simulink subsystem "BATERIA_INVERSOR"  (R2020b)
settings: Solver=VariableStepAuto  StartTime=0.0  StopTime=10.0  RelTol=1e-3
undefined symbols (not defined in the file): Ion, Lithium, Ts
libraries: powerlib x34, powerlib_meascontrol x11, slpidlib x11, electricdrivelib x1, simulink x1
(part 1 of 2)
settings Model: Creator=JGC  LastModifiedBy=JGC

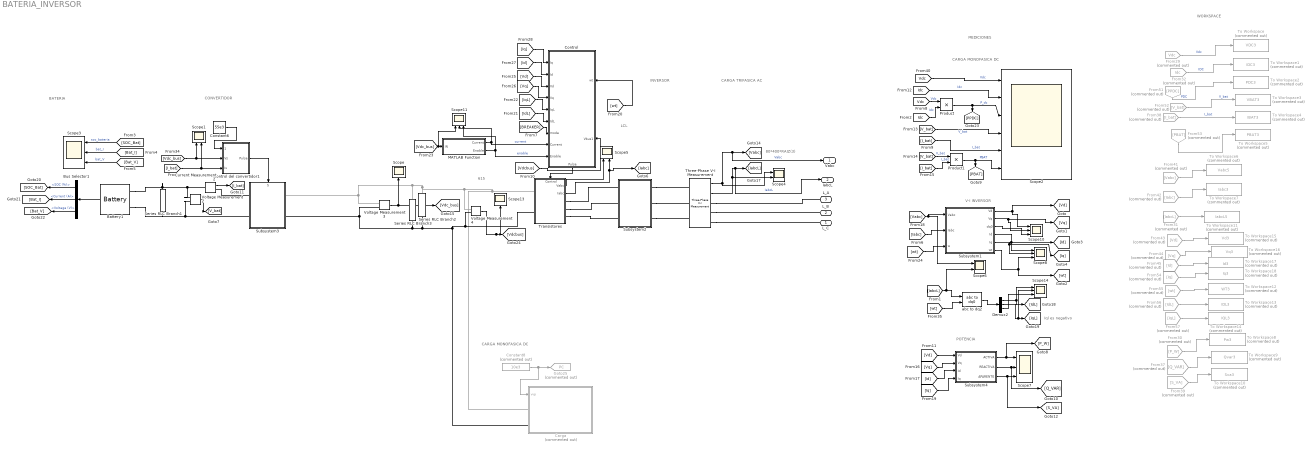
== system BATERIA_INVERSOR ==
  note: CARGA TRIFASICA AC
  note: LCL
  note: CARGA MONOFASICA DC
  note: BATERIA
  note: 80*400*RAIZ(3)
  note: 615
  note: CONVERTIDOR
  note: INVERSOR
  note: Iql es negativo
  note: V-I INVERSOR
  note: MEDICIONES
  note: CARGA MONOFASICA DC
  note: POTENCIA
  note: WORKSPACE
  Battery1 : electricdrivelib/Extra Sources/Battery  BatType=Lithium-Ion  ShowTempParam=off  ThermalPreset=no  ShowAgeParam=off  NomV=Battery.Nominal_voltage  NomQ=Battery.Rated_capacity  SOC=Battery.inicial_state_of_charge  Batt_Tr=Battery.response_time  PresetModel=on  MaxQ=200  MinV=384  FullV=595.9614  Dis_rate=86.9565  R=0.0256  Normal_OP=180.8696  expZone="[553.1576      9.826087]"  current=[6.5 7 100]  Units=Time  Tci=20  NomT=20  T2=-30  MaxQ2=4.8  FullV2=7.1  Normal_OP2=5.655  expZone2="[6.58           1]"  Rca=0.6  ti=2000  Dp=0  Neq0=0  Tsim=1e6  Ta1=25  Qeol=5.4*0.9  Reol=0.013333*1.2  Char_age=[2.3478, 3]  Dis_age=[2.3478, 10]  N1=1500  N2=10500  N3=1000  N4=1400  Ta2=45  N5=950
  Bus Selector1 : BusSelector  OutputSignals=SOC (%),Current (A),Voltage (V)
  Carga : Subsystem  Commented=on
  Constant6 : Constant  Value=55e3
  Constant8 : Constant  Commented=on  Value=10e3
  "Control " : Subsystem
      settings: PortSchema="{\"entries\":[{\"content\":{\"sides\":[{\"content\":{\"connectorIds\":[\"In1\",\"In2\",\"In3\",\"In4\",\"In5\",\"In6\",\"In7\",\"In8\",\"In9\"]},\"type\":\"ConnectorPlacement.EquallySpacedRectSide\",\"uuid\":\"040f479b-0063-4a97-945a-b7b76c14ccf9\"},{\"content\":{\"connectorIds\":[\"In10\",\"In11\"],\"side\":\"RIGHT\"},\"type\":\"ConnectorPlacement.EquallySpacedRectSide\",\"uuid\":\"48d15187-e0ba-47e4-acd1-e370322fb20d\"},{\"content\":{\"connectorIds\":[],\"side\":\"TOP\"},\"type\":\"ConnectorPlacement.EquallySpacedRectSide\",\"uuid\":\"c47ff363-741e-4c95-9660-92ffbbf0858a\"},{\"content\":{\"connectorIds\":[\"Out1\"],\"side\":\"BOTTOM\"},\"type\":\"ConnectorPlacement.EquallySpacedRectSide\",\"uuid\":\"eb550659-5dfa-48af-9c5b-3062ad81491f\"},{\"content\":{\"connectorIds\":[],\"side\":\"HIDDEN\"},\"type\":\"ConnectorPlacement.EquallySpacedRectSide\",\"uuid\":\"d4fe4439-474c-44ef-b2aa-466a1c380da3\"}]},\"type\":\"ConnectorPlacement.EquallySpacedConnector\",\"uuid\":\"b4b94fd9-d3fa-4033-a0eb-720d35d74a7d\"}],\"packageUris\":[\"http://schema.mathworks.com/mf0/Connector/R2020b\"],\"version\":\"1.0\"}"
  Control del convertidor1 : Subsystem
  Current Measurement2 : powerlib/Measurements/Current Measurement  PhasorSimulation=off  OutputType=Complex  PSBequivalent=0
  Demux2 : Demux  Outputs=3
  From29 : From  Commented=on  GotoTag=Vdc
  From30 : From  Commented=on  GotoTag=P_W
  From31 : From  Commented=on  GotoTag=IabcL
  From32 : From  Commented=on  GotoTag=Idc
  From37 : From  Commented=on  GotoTag=Q_VAR
  From38 : From  Commented=on  GotoTag=I_bat
  From39 : From  Commented=on  GotoTag=S_VA
  From41 : From  Commented=on  GotoTag=Vabc
  From42 : From  Commented=on  GotoTag=Iabc
  From43 : From  Commented=on  GotoTag=Vd
  From44 : From  Commented=on  GotoTag=Vq
  From45 : From  Commented=on  GotoTag=Id
  From51 : From  Commented=on  GotoTag=PPDC
  From52 : From  Commented=on  GotoTag=V_bat
  From53 : From  Commented=on  GotoTag=PBAT
  From54 : From  Commented=on  GotoTag=Iq
  From55 : From  Commented=on  GotoTag=wt
  From56 : From  Commented=on  GotoTag=IdL
  From57 : From  Commented=on  GotoTag=IqL
  Goto25 : Goto  Commented=on  GotoTag=PC  TagVisibility=global
  MATLAB Function : MATLAB Function  TreatAsAtomicUnit=on
  Product : Product
  Product1 : Product
  Scope : Scope
  Scope{1,4..6} (4 alike) : Scope  NumInputPorts=2
  Scope{3,7..8,10..11,14} (6 alike) : Scope  NumInputPorts=3
  Scope13 : Scope
  Scope2 : Scope  NumInputPorts=6
  Series RLC Branch1 : powerlib/Elements/Series RLC Branch  LConnTagsString=__new0  RConnTagsString=__new0  BranchType=RC  Resistance=0.3  Inductance=1e-3  SetiL0=off  InitialCurrent=0  Capacitance=1e-6  Setx0=on  InitialVoltage=512  Measurements=None
  Series RLC Branch2 : powerlib/Elements/Series RLC Branch  LConnTagsString=__new0  RConnTagsString=__new0  BranchType=C  Resistance=0.2  Inductance=1e-3  SetiL0=off  InitialCurrent=0  Capacitance=1000e-6  Setx0=on  InitialVoltage=550  Measurements=None
  Series RLC Branch3 : powerlib/Elements/Series RLC Branch  LConnTagsString=__new0  RConnTagsString=__new0  BranchType=R  Resistance=38  Inductance=1e-3  SetiL0=off  InitialCurrent=0  Capacitance=1e-6  Setx0=on  InitialVoltage=512  Measurements=None
  Subsystem1 : Subsystem
  Subsystem2 : Subsystem
  Subsystem3 : Subsystem
      settings: PortSchema="{\"entries\":[{\"content\":{\"sides\":[{\"content\":{\"connectorIds\":[\"LConn1\",\"LConn2\"]},\"type\":\"ConnectorPlacement.EquallySpacedRectSide\",\"uuid\":\"7a980847-0fd3-4a52-ae22-59cd2a1ed559\"},{\"content\":{\"connectorIds\":[\"RConn1\",\"RConn2\"],\"side\":\"RIGHT\"},\"type\":\"ConnectorPlacement.EquallySpacedRectSide\",\"uuid\":\"85effeeb-73a6-4b0a-b51b-5eb0082317ff\"},{\"content\":{\"connectorIds\":[\"In1\"],\"side\":\"TOP\"},\"type\":\"ConnectorPlacement.EquallySpacedRectSide\",\"uuid\":\"eb55fae0-79ad-414f-ab96-49c332138803\"},{\"content\":{\"connectorIds\":[],\"side\":\"BOTTOM\"},\"type\":\"ConnectorPlacement.EquallySpacedRectSide\",\"uuid\":\"1fd972ff-419a-4657-8ea4-57d89be2b868\"}]},\"type\":\"ConnectorPlacement.EquallySpacedConnector\",\"uuid\":\"1807473d-fd42-44e0-a7e4-668a7bf21429\"}],\"packageUris\":[\"http://schema.mathworks.com/mf0/Connector/R2020b\"],\"version\":\"1.0\"}"
  Subsystem4 : Subsystem
  Three-Phase V-I Measurement : powerlib/Measurements/Three-Phase V-I Measurement  VoltageMeasurement=phase-to-phase  SetLabelV=off  LabelV=Vabc  Vpu=off  VpuLL=off  CurrentMeasurement=yes  SetLabelI=off  LabelI=Iabc  Ipu=off  Pbase=100e6  Vbase=500e3  OutputType=Complex  PhasorSimulation=off  PSBequivalent=0
  To Workspace : ToWorkspace  Commented=on  VariableName=VDC3  SaveFormat=Timeseries  SampleTime=-1
  To Workspace1 : ToWorkspace  Commented=on  VariableName=IDC3  SaveFormat=Timeseries  SampleTime=-1
  To Workspace10 : ToWorkspace  Commented=on  VariableName=Sva3  SaveFormat=Timeseries  SampleTime=-1
  To Workspace11 : ToWorkspace  Commented=on  VariableName=IabcL5  SaveFormat=Structure With Time  SampleTime=-1
  To Workspace12 : ToWorkspace  Commented=on  VariableName=WT3  SaveFormat=Timeseries  SampleTime=-1
  To Workspace13 : ToWorkspace  Commented=on  VariableName=IDL3  SaveFormat=Timeseries  SampleTime=-1
  To Workspace14 : ToWorkspace  Commented=on  VariableName=IQL3  SaveFormat=Timeseries  SampleTime=-1
  To Workspace15 : ToWorkspace  Commented=on  VariableName=Vd3  SaveFormat=Timeseries  SampleTime=-1
  To Workspace16 : ToWorkspace  Commented=on  VariableName=Vq3  SaveFormat=Timeseries  SampleTime=-1
  To Workspace17 : ToWorkspace  Commented=on  VariableName=Id3  SaveFormat=Timeseries  SampleTime=-1
  To Workspace18 : ToWorkspace  Commented=on  VariableName=Iq3  SaveFormat=Timeseries  SampleTime=-1
  To Workspace2 : ToWorkspace  Commented=on  VariableName=PDC3  SaveFormat=Timeseries  SampleTime=-1
  To Workspace3 : ToWorkspace  Commented=on  VariableName=VBAT3  SaveFormat=Timeseries  SampleTime=-1
  To Workspace4 : ToWorkspace  Commented=on  VariableName=IBAT3  SaveFormat=Timeseries  SampleTime=-1
  To Workspace5 : ToWorkspace  Commented=on  VariableName=PBAT3  SaveFormat=Timeseries  SampleTime=-1
  To Workspace6 : ToWorkspace  Commented=on  VariableName=Vabc5  SaveFormat=Structure With Time  SampleTime=-1
  To Workspace7 : ToWorkspace  Commented=on  VariableName=Iabc3  SaveFormat=Timeseries  SampleTime=-1
  To Workspace8 : ToWorkspace  Commented=on  VariableName=Pw3  SaveFormat=Timeseries  SampleTime=-1
  To Workspace9 : ToWorkspace  Commented=on  VariableName=Qvar3  SaveFormat=Timeseries  SampleTime=-1
  Transistores : Subsystem
      settings: PortSchema="{\"entries\":[{\"content\":{\"sides\":[{\"content\":{\"connectorIds\":[\"LConn1\",\"LConn2\"]},\"type\":\"ConnectorPlacement.EquallySpacedRectSide\",\"uuid\":\"4b4a90af-a54c-4879-a767-640ef5f3fcb3\"},{\"content\":{\"connectorIds\":[\"Out1\",\"Out2\",\"RConn1\",\"RConn2\",\"RConn3\"],\"side\":\"RIGHT\"},\"type\":\"ConnectorPlacement.EquallySpacedRectSide\",\"uuid\":\"9175716d-9f9b-4229-800b-ed18d0bc4919\"},{\"content\":{\"connectorIds\":[\"In1\"],\"side\":\"TOP\"},\"type\":\"ConnectorPlacement.EquallySpacedRectSide\",\"uuid\":\"ad8bb3e4-0cf0-4c72-aeb3-553776322e14\"},{\"content\":{\"connectorIds\":[],\"side\":\"HIDDEN\"},\"type\":\"ConnectorPlacement.EquallySpacedRectSide\",\"uuid\":\"389b5ba2-67e8-44c1-bbe9-0320a382984d\"}]},\"type\":\"ConnectorPlacement.EquallySpacedConnector\",\"uuid\":\"7a2ee168-b262-4afb-be64-1e845efa873f\"}],\"packageUris\":[\"http://schema.mathworks.com/mf0/Connector/R2020b\"],\"version\":\"1.0\"}"
  Voltage Measurement2 : powerlib/Measurements/Voltage Measurement  PhasorSimulation=off  OutputType=Complex  PSBequivalent=0
  Voltage Measurement3 : powerlib/Measurements/Voltage Measurement  PhasorSimulation=off  OutputType=Complex  PSBequivalent=0
  Voltage Measurement4 : powerlib/Measurements/Voltage Measurement  PhasorSimulation=off  OutputType=Complex  PSBequivalent=0
  abc to dq2 : powerlib_meascontrol/Transformations/abc to dq0  Alignment=90 degrees behind phase A axis
  L_C : PMIOPort  Side=Right
  L_B : PMIOPort  Port=2  Side=Right
  L_A : PMIOPort  Port=3  Side=Right
  Vabc : Outport
  IabcL : Outport  Port=2
  wires:
  Current Measurement2/1 -> [I_bat]
  Voltage Measurement2/1 -> [V_bat]
  Transistores/1(Vabc) -> Scope5/1
  Control del convertidor1/1(Pulse) -> Subsystem3/1(S)
  [Bat_V] -> Scope3/3  "bat_V"
  Transistores/2(Iabc) -> Scope5/2, [Iabc]
  Three-Phase V-I Measurement/2 -> Scope4/2, [IabcL], IabcL/1  "IabcL"
  Constant6/1 -> Control del convertidor1/1(Pot_ref)
  [Bat_I] -> Scope3/2  "bat_I"
  Three-Phase V-I Measurement/1 -> Scope4/1, [Vabc], Vabc/1  "Vabc"
  "Control "/1(Pulse) -> Transistores/1(Control)
  MATLAB Function/2(Enable) -> "Control "/9(Enable), Scope11/3  "enable"
  Battery1/1 -> Bus Selector1/1
  [Vdc_bus] -> Control del convertidor1/2(Vs), Scope1/1
  [I_bat] -> Scope1/2, Control del convertidor1/3(Is)
  MATLAB Function/1(Current) -> "Control "/8(Current), Scope11/2  "current"
  Bus Selector1/2 -> [Bat_I]  "<Current (A)>"
  Constant8/1 -> Carga/1(vvp), Goto25/1
  Bus Selector1/1 -> [SOC_Bat]  "<SOC (%)>"
  Voltage Measurement3/1 -> Scope/1, [Vdc_bus]
  [SOC_Bat] -> Scope3/1  "soc_bateria"
  Bus Selector1/3 -> [Bat_V]  "<Voltage (V)>"
  Voltage Measurement4/1 -> [Vdcbus], Scope13/1
  [Vdc_bus] -> MATLAB Function/1(IN), Scope11/1
  [Vdcbus] -> "Control "/11(Vbus1)
  [BREAKER] -> "Control "/7(mode)
  Demux2/1 -> Scope14/1, [IdL]
  [I_bat] -> Product1/2  "I_bat"
  [I_bat] -> Scope2/5  "I_bat"
  Demux2/2 -> [IqL], Scope14/2
  Subsystem1/2(Vq) -> [Vq], Scope10/2
  abc to dq2/1 -> Demux2/1
  [Vdc] -> Scope2/1  "Vdc"
  Subsystem4/1(ACTIVA) -> Scope7/1, [P_W]
  [Idc] -> Scope2/2  "Idc"
  Subsystem1/5(Iq) -> [Iq], Scope8/2
  [V_bat] -> Product1/1  "V_bat"
  [IabcL] -> abc to dq2/1, Scope6/2
  [V_bat] -> Scope2/4  "V_bat"
  Subsystem1/6(wt) -> Scope8/3, [wt]
  [Vdc] -> Product/1  "Vdc"
  Product1/1 -> [PBAT], Scope2/6  "PBAT"
  [Iabc] -> Subsystem1/2(Iabc)
  Subsystem1/1(Vd) -> [Vd], Scope10/1
  Product/1 -> [PPDC], Scope2/3  "P_dc"
  [wt] -> abc to dq2/2
  [Idc] -> Product/2  "Idc"
  Subsystem1/4(Id) -> Scope8/1, [Id]
  Demux2/3 -> Scope14/3
  [Vabc] -> Subsystem1/1(Vabc), Scope6/1
  Subsystem4/3(APARENTE) -> Scope7/3, [S_VA]
  Subsystem1/3(dq0) -> Scope10/3
  Subsystem4/2(REACTIVA) -> Scope7/2, [Q_VAR]
  [Vd] -> Subsystem4/1(Vd)
  [Vq] -> Subsystem4/2(Vq)
  [Id] -> Subsystem4/3(Id)
  [Iq] -> Subsystem4/4(Iq)
  [wt] -> "Control "/10(wt)
  [IdL] -> "Control "/6(IdL)
  [IqL] -> "Control "/5(IqL)
  [wt] -> Subsystem1/3(w)
  [Vd] -> "Control "/3(Vd)
  [Vq] -> "Control "/4(Vq)
  [Id] -> "Control "/2(Id)
  [Iq] -> "Control "/1(Iq)
  From56/1 -> To Workspace13/1
  From45/1 -> To Workspace17/1
  From31/1 -> To Workspace11/1
  From54/1 -> To Workspace18/1
  From51/1 -> To Workspace2/1  "PDC"
  From39/1 -> To Workspace10/1
  From43/1 -> To Workspace15/1
  From53/1 -> To Workspace5/1
  From52/1 -> To Workspace3/1  "V_bat"
  From37/1 -> To Workspace9/1
  From41/1 -> To Workspace6/1
  From42/1 -> To Workspace7/1
  From38/1 -> To Workspace4/1  "I_bat"
  From57/1 -> To Workspace14/1
  From29/1 -> To Workspace/1  "Vdc"
  From30/1 -> To Workspace8/1
  From32/1 -> To Workspace1/1  "IDC"
  From55/1 -> To Workspace12/1
  From44/1 -> To Workspace16/1
  connections:
  Carga/LConn1 -- Voltage Measurement3/LConn1 -- Subsystem3/RConn1 -- Series RLC Branch3/LConn1 -- Series RLC Branch2/LConn1 -- Voltage Measurement4/LConn1 -- Transistores/LConn1
  Series RLC Branch1/LConn1 -- Current Measurement2/LConn1 -- Voltage Measurement2/LConn1 -- Battery1/LConn1
  Transistores/LConn2 -- Voltage Measurement3/LConn2 -- Subsystem3/RConn2 -- Series RLC Branch3/RConn1 -- Series RLC Branch2/RConn1 -- Carga/LConn2 -- Voltage Measurement4/LConn2
  Subsystem3/LConn2 -- Series RLC Branch1/RConn1 -- Battery1/LConn2 -- Voltage Measurement2/LConn2
  Subsystem3/LConn1 -- Current Measurement2/RConn1
  Three-Phase V-I Measurement/RConn2 -- L_B/RConn1
  Subsystem2/LConn2 -- Three-Phase V-I Measurement/LConn2
  Three-Phase V-I Measurement/RConn1 -- L_A/RConn1
  Three-Phase V-I Measurement/RConn3 -- L_C/RConn1
  Transistores/RConn2 -- Subsystem2/RConn2
  Subsystem2/LConn3 -- Three-Phase V-I Measurement/LConn3
  Subsystem2/LConn1 -- Three-Phase V-I Measurement/LConn1
  Transistores/RConn3 -- Subsystem2/RConn3
  Transistores/RConn1 -- Subsystem2/RConn1

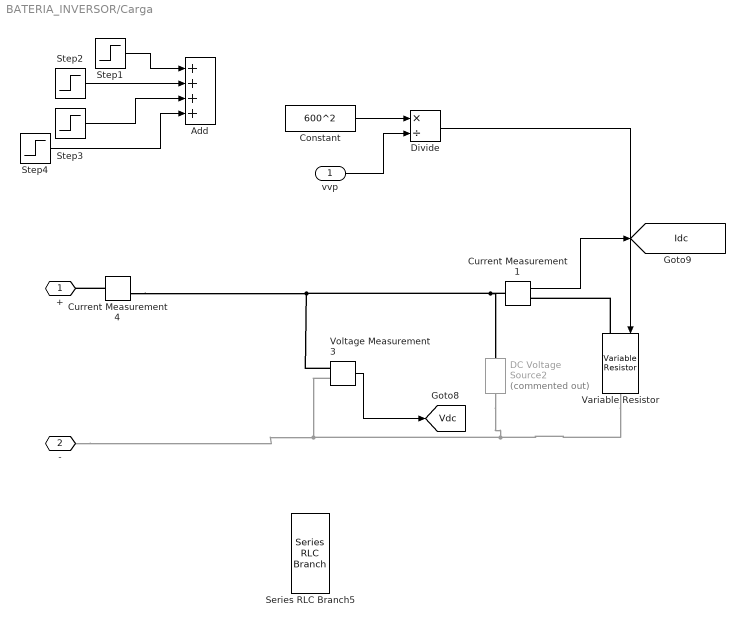
== system BATERIA_INVERSOR/Carga ==
  vvp : Inport
  Add : Sum  Inputs=++++
  Constant : Constant  Value=600^2
  Current Measurement1 : powerlib/Measurements/Current Measurement  PhasorSimulation=off  OutputType=Complex  PSBequivalent=0
  Current Measurement4 : powerlib/Measurements/Current Measurement  PhasorSimulation=off  OutputType=Complex  PSBequivalent=0
  DC Voltage Source2 : powerlib/Electrical Sources/DC Voltage Source  Commented=on  Amplitude=800  Measurements=None
  Divide : Product  Inputs=*/
  Series RLC Branch5 : powerlib/Elements/Series RLC Branch  LConnTagsString=__new0  RConnTagsString=__new0  BranchType=C  Resistance=0.2  Inductance=1e-3  SetiL0=off  InitialCurrent=0  Capacitance=300e-6  Setx0=on  InitialVoltage=512  Measurements=None
  Step1 : Step  After=5000  SampleTime=0
  Step2 : Step  Time=2  After=-7500  SampleTime=0
  Step3 : Step  Time=3  After=10000  SampleTime=0
  Step4 : Step  Time=4  After=-7500  SampleTime=0
  Variable Resistor : powerlib/Elements/Variable Resistor  Rabsmin=1e-3
      settings: SourceProductBaseCode=PS
  Voltage Measurement3 : powerlib/Measurements/Voltage Measurement  PhasorSimulation=off  OutputType=Complex  PSBequivalent=0
  + : PMIOPort  Side=Left
  - : PMIOPort  Port=2  Side=Left
  tag scope: Idc=global, Vdc=global
  wires:
  vvp/1 -> Divide/2
  Current Measurement1/1 -> [Idc]
  Step4/1 -> Add/4
  Step3/1 -> Add/3
  Step2/1 -> Add/2
  Step1/1 -> Add/1
  Divide/1 -> Variable Resistor/1
  Constant/1 -> Divide/1
  Voltage Measurement3/1 -> [Vdc]
  connections:
  Current Measurement1/LConn1 -- DC Voltage Source2/RConn1 -- Voltage Measurement3/LConn1 -- Current Measurement4/RConn1
  Variable Resistor/LConn1 -- Current Measurement1/RConn1
  Current Measurement4/LConn1 -- +/RConn1
  DC Voltage Source2/LConn1 -- Variable Resistor/RConn1 -- -/RConn1 -- Voltage Measurement3/LConn2

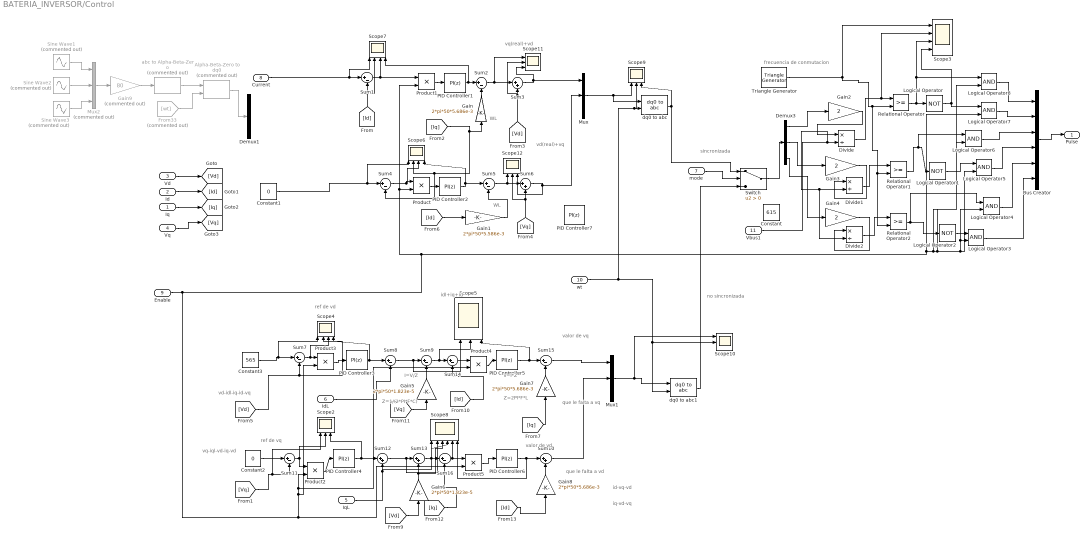
== system BATERIA_INVERSOR/Control  ==
  note: v=I*Z
  note: Z=2PI*F*L
  note: vd-idl-iq-id-vq
  note: ref de vq
  note: que le falta a vd
  note: ref de vd
  note: que le falta a vq
  note: valor de vq
  note: iq-vd-vq
  note: valor de vd
  note: vq-iql-vd-iq-vd
  note: I=V/Z
  note: Z=1/(2*PI*F*C)
  note: id-vq-vd
  note: idl+iq+id
  note: vq(real)+vd
  note: vd(real)+vq
  note: WL
  note: WL
  note: frecuencia de conmutacion
  note: no sincronizada
  note: sincronizada
  Iq : Inport
  Id : Inport  Port=2
  Vd : Inport  Port=3
  Vq : Inport  Port=4
  IqL : Inport  Port=5
  IdL : Inport  Port=6
  mode : Inport  Port=7
  Current : Inport  Port=8
  Enable : Inport  Port=9
  wt : Inport  Port=10
  Vbus1 : Inport  Port=11
  Alpha-Beta-Zero to dq0 : powerlib_meascontrol/Transformations/Alpha-Beta-Zero to dq0  Commented=on  Alignment=90 degrees behind phase A axis
  Bus Creator : BusCreator  Inputs=6
  Constant : Constant  Value=615
  Constant1 : Constant  Value=0
  Constant2 : Constant  Value=0
  Constant3 : Constant  Value=565
  Demux1 : Demux  Outputs=3
  Demux3 : Demux  Outputs=3
  Divide : Product  Inputs=*/
  Divide1 : Product  Inputs=*/
  Divide2 : Product  Inputs=*/
  From33 : From  Commented=on  GotoTag=wt  TagVisibility=global
  Gain : Gain  Gain=2*pi*50*5.686e-3
  Gain1 : Gain  Gain=2*pi*50*5.586e-3
  Gain2 : Gain  Gain=2
  Gain3 : Gain  Gain=2
  Gain4 : Gain  Gain=2
  Gain5 : Gain  Gain=2*pi*50*1.823e-5
  Gain6 : Gain  Gain=2*pi*50*1.823e-5
  Gain7 : Gain  Gain=2*pi*50*5.686e-3
  Gain8 : Gain  Gain=2*pi*50*5.686e-3
  Gain9 : Gain  Commented=on  Gain=80
  Logical Operator : Logic  Operator=NOT  AllPortsSameDT=off  OutDataTypeStr=boolean
  Logical Operator1 : Logic  Operator=NOT  AllPortsSameDT=off  OutDataTypeStr=boolean
  Logical Operator2 : Logic  Operator=NOT  AllPortsSameDT=off  OutDataTypeStr=boolean
  Logical Operator{3..8} (6 alike) : Logic  AllPortsSameDT=off  OutDataTypeStr=boolean
  Mux : Mux  Inputs=3
  Mux1 : Mux  Inputs=3
  Mux2 : Mux  Commented=on  Inputs=3
  PID Controller1 : slpidlib/PID Controller  Controller=PI  Form=Parallel  TimeDomain=Discrete-time  UseExternalTs=off  SampleTime=Ts  IntegratorMethod=Forward Euler  FilterMethod=Forward Euler  ControllerParametersSource=internal  P=60  I=0  D=0  UseFilter=on  N=100  TunerSelectOption=Transfer Function Based (PID Tuner App)  InitialConditionSource=internal  InitialConditionForIntegrator=0  InitialConditionForFilter=0  DifferentiatorICPrevScaledInput=0  ExternalReset=none  TrackingMode=off  Kt=1  LimitOutput=off  SatLimitsSource=internal  UpperSaturationLimit=inf  LowerSaturationLimit=-inf  LinearizeAsGain=on  AntiWindupMode=none  Kb=1  POutMin=[]  POutMax=[]  IOutMin=[]  IOutMax=[]  DOutMin=[]  DOutMax=[]  NOutMin=[]  NOutMax=[]  SumOutMin=[]  SumOutMax=[]  SaturationOutMin=[]  SaturationOutMax=[]  PParamMin=[]  PParamMax=[]  IParamMin=[]  IParamMax=[]  DParamMin=[]  DParamMax=[]  NParamMin=[]  NParamMax=[]  KbParamMin=[]  KbParamMax=[]  KtParamMin=[]  KtParamMax=[]  KbOutMin=[]  KbOutMax=[]  KtOutMin=[]  KtOutMax=[]  IntegratorOutMin=[]  IntegratorOutMax=[]  FilterOutMin=[]  FilterOutMax=[]  SumI1OutMin=[]  SumI1OutMax=[]  SumI2OutMin=[]  SumI2OutMax=[]  SumI3OutMin=[]  SumI3OutMax=[]  SumI4OutMin=[]  SumI4OutMax=[]  SumDOutMin=[]  SumDOutMax=[]  DifferentiatorOutMin=[]  DifferentiatorOutMax=[]  FilterDiffOutCoefMin=[]  FilterDiffOutCoefMax=[]  ReciprocalOutMin=[]  ReciprocalOutMax=[]  SumDenOutMin=[]  SumDenOutMax=[]  SumNumOutMin=[]  SumNumOutMax=[]  DivideOutMin=[]  DivideOutMax=[]  UdiffTsProdOutMin=[]  UdiffTsProdOutMax=[]  NTsProdOutMin=[]  NTsProdOutMax=[]  UintegralTsProdOutMin=[]  UintegralTsProdOutMax=[]  UngainTsProdOutMin=[]  UngainTsProdOutMax=[]  IntegratorContinuousStateAttributes=''  IntegratorStateMustResolveToSignalObject=off  IntegratorRTWStateStorageClass=Auto  FilterContinuousStateAttributes=''  FilterStateMustResolveToSignalObject=off  FilterRTWStateStorageClass=Auto  ParallelPVariant=InternalParameters  IdealPVariant=Disabled  IVariant=InternalParameters  DVariant=Disabled  IntegratorVariant=Discrete  SatVariant=Disabled  AWVariant=Passthrough  PCopyVariant=Disabled  TRVariant=Disabled  FdbkBlocksVariant=Forward  IdealPFdbkVariant=Disabled  SatFdbkVariant=Disabled  DerivativeFilterVariant=Disabled  NVariant=Disabled  NCopyVariant=Disabled_SignalSpec  FilterICVariant=Disabled  IntegratorICVariant=InternalICs  ExternalResetVariant=Disabled  TRSumVariant=Passthrough  SumFdbkVariant=Disabled  SumVariant=Sum_PI  TsampFilterVariant=InternalTs  TsampNgainVariant=Passthrough  TsampIntegralVariant=Passthrough  ExternalSaturationOutDataTypeStr=Inherit: Same as second input
  PID Controller2 : slpidlib/PID Controller  Controller=PI  Form=Parallel  TimeDomain=Discrete-time  UseExternalTs=off  SampleTime=Ts  IntegratorMethod=Forward Euler  FilterMethod=Forward Euler  ControllerParametersSource=internal  P=70  I=10  D=0  UseFilter=on  N=100  TunerSelectOption=Transfer Function Based (PID Tuner App)  InitialConditionSource=internal  InitialConditionForIntegrator=0  InitialConditionForFilter=0  DifferentiatorICPrevScaledInput=0  ExternalReset=none  TrackingMode=off  Kt=1  LimitOutput=off  SatLimitsSource=internal  UpperSaturationLimit=inf  LowerSaturationLimit=-inf  LinearizeAsGain=on  AntiWindupMode=none  Kb=1  POutMin=[]  POutMax=[]  IOutMin=[]  IOutMax=[]  DOutMin=[]  DOutMax=[]  NOutMin=[]  NOutMax=[]  SumOutMin=[]  SumOutMax=[]  SaturationOutMin=[]  SaturationOutMax=[]  PParamMin=[]  PParamMax=[]  IParamMin=[]  IParamMax=[]  DParamMin=[]  DParamMax=[]  NParamMin=[]  NParamMax=[]  KbParamMin=[]  KbParamMax=[]  KtParamMin=[]  KtParamMax=[]  KbOutMin=[]  KbOutMax=[]  KtOutMin=[]  KtOutMax=[]  IntegratorOutMin=[]  IntegratorOutMax=[]  FilterOutMin=[]  FilterOutMax=[]  SumI1OutMin=[]  SumI1OutMax=[]  SumI2OutMin=[]  SumI2OutMax=[]  SumI3OutMin=[]  SumI3OutMax=[]  SumI4OutMin=[]  SumI4OutMax=[]  SumDOutMin=[]  SumDOutMax=[]  DifferentiatorOutMin=[]  DifferentiatorOutMax=[]  FilterDiffOutCoefMin=[]  FilterDiffOutCoefMax=[]  ReciprocalOutMin=[]  ReciprocalOutMax=[]  SumDenOutMin=[]  SumDenOutMax=[]  SumNumOutMin=[]  SumNumOutMax=[]  DivideOutMin=[]  DivideOutMax=[]  UdiffTsProdOutMin=[]  UdiffTsProdOutMax=[]  NTsProdOutMin=[]  NTsProdOutMax=[]  UintegralTsProdOutMin=[]  UintegralTsProdOutMax=[]  UngainTsProdOutMin=[]  UngainTsProdOutMax=[]  IntegratorContinuousStateAttributes=''  IntegratorStateMustResolveToSignalObject=off  IntegratorRTWStateStorageClass=Auto  FilterContinuousStateAttributes=''  FilterStateMustResolveToSignalObject=off  FilterRTWStateStorageClass=Auto  ParallelPVariant=InternalParameters  IdealPVariant=Disabled  IVariant=InternalParameters  DVariant=Disabled  IntegratorVariant=Discrete  SatVariant=Disabled  AWVariant=Passthrough  PCopyVariant=Disabled  TRVariant=Disabled  FdbkBlocksVariant=Forward  IdealPFdbkVariant=Disabled  SatFdbkVariant=Disabled  DerivativeFilterVariant=Disabled  NVariant=Disabled  NCopyVariant=Disabled_SignalSpec  FilterICVariant=Disabled  IntegratorICVariant=InternalICs  ExternalResetVariant=Disabled  TRSumVariant=Passthrough  SumFdbkVariant=Disabled  SumVariant=Sum_PI  TsampFilterVariant=InternalTs  TsampNgainVariant=Passthrough  TsampIntegralVariant=Passthrough  ExternalSaturationOutDataTypeStr=Inherit: Same as second input
  PID Controller3 : slpidlib/PID Controller  Controller=PI  Form=Parallel  TimeDomain=Discrete-time  UseExternalTs=off  SampleTime=Ts  IntegratorMethod=Forward Euler  FilterMethod=Forward Euler  ControllerParametersSource=internal  P=1  I=180  D=0  UseFilter=on  N=100  TunerSelectOption=Transfer Function Based (PID Tuner App)  InitialConditionSource=internal  InitialConditionForIntegrator=0  InitialConditionForFilter=0  DifferentiatorICPrevScaledInput=0  ExternalReset=none  TrackingMode=off  Kt=1  LimitOutput=off  SatLimitsSource=internal  UpperSaturationLimit=inf  LowerSaturationLimit=-inf  LinearizeAsGain=on  AntiWindupMode=none  Kb=1  POutMin=[]  POutMax=[]  IOutMin=[]  IOutMax=[]  DOutMin=[]  DOutMax=[]  NOutMin=[]  NOutMax=[]  SumOutMin=[]  SumOutMax=[]  SaturationOutMin=[]  SaturationOutMax=[]  PParamMin=[]  PParamMax=[]  IParamMin=[]  IParamMax=[]  DParamMin=[]  DParamMax=[]  NParamMin=[]  NParamMax=[]  KbParamMin=[]  KbParamMax=[]  KtParamMin=[]  KtParamMax=[]  KbOutMin=[]  KbOutMax=[]  KtOutMin=[]  KtOutMax=[]  IntegratorOutMin=[]  IntegratorOutMax=[]  FilterOutMin=[]  FilterOutMax=[]  SumI1OutMin=[]  SumI1OutMax=[]  SumI2OutMin=[]  SumI2OutMax=[]  SumI3OutMin=[]  SumI3OutMax=[]  SumI4OutMin=[]  SumI4OutMax=[]  SumDOutMin=[]  SumDOutMax=[]  DifferentiatorOutMin=[]  DifferentiatorOutMax=[]  FilterDiffOutCoefMin=[]  FilterDiffOutCoefMax=[]  ReciprocalOutMin=[]  ReciprocalOutMax=[]  SumDenOutMin=[]  SumDenOutMax=[]  SumNumOutMin=[]  SumNumOutMax=[]  DivideOutMin=[]  DivideOutMax=[]  UdiffTsProdOutMin=[]  UdiffTsProdOutMax=[]  NTsProdOutMin=[]  NTsProdOutMax=[]  UintegralTsProdOutMin=[]  UintegralTsProdOutMax=[]  UngainTsProdOutMin=[]  UngainTsProdOutMax=[]  IntegratorContinuousStateAttributes=''  IntegratorStateMustResolveToSignalObject=off  IntegratorRTWStateStorageClass=Auto  FilterContinuousStateAttributes=''  FilterStateMustResolveToSignalObject=off  FilterRTWStateStorageClass=Auto  ParallelPVariant=InternalParameters  IdealPVariant=Disabled  IVariant=InternalParameters  DVariant=Disabled  IntegratorVariant=Discrete  SatVariant=Disabled  AWVariant=Passthrough  PCopyVariant=Disabled  TRVariant=Disabled  FdbkBlocksVariant=Forward  IdealPFdbkVariant=Disabled  SatFdbkVariant=Disabled  DerivativeFilterVariant=Disabled  NVariant=Disabled  NCopyVariant=Disabled_SignalSpec  FilterICVariant=Disabled  IntegratorICVariant=InternalICs  ExternalResetVariant=Disabled  TRSumVariant=Passthrough  SumFdbkVariant=Disabled  SumVariant=Sum_PI  TsampFilterVariant=InternalTs  TsampNgainVariant=Passthrough  TsampIntegralVariant=Passthrough  ExternalSaturationOutDataTypeStr=Inherit: Same as second input
  PID Controller4 : slpidlib/PID Controller  Controller=PI  Form=Parallel  TimeDomain=Discrete-time  UseExternalTs=off  SampleTime=Ts  IntegratorMethod=Forward Euler  FilterMethod=Forward Euler  ControllerParametersSource=internal  P=1  I=180  D=0  UseFilter=on  N=100  TunerSelectOption=Transfer Function Based (PID Tuner App)  InitialConditionSource=internal  InitialConditionForIntegrator=0  InitialConditionForFilter=0  DifferentiatorICPrevScaledInput=0  ExternalReset=none  TrackingMode=off  Kt=1  LimitOutput=off  SatLimitsSource=internal  UpperSaturationLimit=inf  LowerSaturationLimit=-inf  LinearizeAsGain=on  AntiWindupMode=none  Kb=1  POutMin=[]  POutMax=[]  IOutMin=[]  IOutMax=[]  DOutMin=[]  DOutMax=[]  NOutMin=[]  NOutMax=[]  SumOutMin=[]  SumOutMax=[]  SaturationOutMin=[]  SaturationOutMax=[]  PParamMin=[]  PParamMax=[]  IParamMin=[]  IParamMax=[]  DParamMin=[]  DParamMax=[]  NParamMin=[]  NParamMax=[]  KbParamMin=[]  KbParamMax=[]  KtParamMin=[]  KtParamMax=[]  KbOutMin=[]  KbOutMax=[]  KtOutMin=[]  KtOutMax=[]  IntegratorOutMin=[]  IntegratorOutMax=[]  FilterOutMin=[]  FilterOutMax=[]  SumI1OutMin=[]  SumI1OutMax=[]  SumI2OutMin=[]  SumI2OutMax=[]  SumI3OutMin=[]  SumI3OutMax=[]  SumI4OutMin=[]  SumI4OutMax=[]  SumDOutMin=[]  SumDOutMax=[]  DifferentiatorOutMin=[]  DifferentiatorOutMax=[]  FilterDiffOutCoefMin=[]  FilterDiffOutCoefMax=[]  ReciprocalOutMin=[]  ReciprocalOutMax=[]  SumDenOutMin=[]  SumDenOutMax=[]  SumNumOutMin=[]  SumNumOutMax=[]  DivideOutMin=[]  DivideOutMax=[]  UdiffTsProdOutMin=[]  UdiffTsProdOutMax=[]  NTsProdOutMin=[]  NTsProdOutMax=[]  UintegralTsProdOutMin=[]  UintegralTsProdOutMax=[]  UngainTsProdOutMin=[]  UngainTsProdOutMax=[]  IntegratorContinuousStateAttributes=''  IntegratorStateMustResolveToSignalObject=off  IntegratorRTWStateStorageClass=Auto  FilterContinuousStateAttributes=''  FilterStateMustResolveToSignalObject=off  FilterRTWStateStorageClass=Auto  ParallelPVariant=InternalParameters  IdealPVariant=Disabled  IVariant=InternalParameters  DVariant=Disabled  IntegratorVariant=Discrete  SatVariant=Disabled  AWVariant=Passthrough  PCopyVariant=Disabled  TRVariant=Disabled  FdbkBlocksVariant=Forward  IdealPFdbkVariant=Disabled  SatFdbkVariant=Disabled  DerivativeFilterVariant=Disabled  NVariant=Disabled  NCopyVariant=Disabled_SignalSpec  FilterICVariant=Disabled  IntegratorICVariant=InternalICs  ExternalResetVariant=Disabled  TRSumVariant=Passthrough  SumFdbkVariant=Disabled  SumVariant=Sum_PI  TsampFilterVariant=InternalTs  TsampNgainVariant=Passthrough  TsampIntegralVariant=Passthrough  ExternalSaturationOutDataTypeStr=Inherit: Same as second input
  PID Controller5 : slpidlib/PID Controller  Controller=PI  Form=Parallel  TimeDomain=Discrete-time  UseExternalTs=off  SampleTime=Ts  IntegratorMethod=Forward Euler  FilterMethod=Forward Euler  ControllerParametersSource=internal  P=10  I=30  D=0  UseFilter=on  N=100  TunerSelectOption=Transfer Function Based (PID Tuner App)  InitialConditionSource=internal  InitialConditionForIntegrator=0  InitialConditionForFilter=0  DifferentiatorICPrevScaledInput=0  ExternalReset=none  TrackingMode=off  Kt=1  LimitOutput=off  SatLimitsSource=internal  UpperSaturationLimit=inf  LowerSaturationLimit=-inf  LinearizeAsGain=on  AntiWindupMode=none  Kb=1  POutMin=[]  POutMax=[]  IOutMin=[]  IOutMax=[]  DOutMin=[]  DOutMax=[]  NOutMin=[]  NOutMax=[]  SumOutMin=[]  SumOutMax=[]  SaturationOutMin=[]  SaturationOutMax=[]  PParamMin=[]  PParamMax=[]  IParamMin=[]  IParamMax=[]  DParamMin=[]  DParamMax=[]  NParamMin=[]  NParamMax=[]  KbParamMin=[]  KbParamMax=[]  KtParamMin=[]  KtParamMax=[]  KbOutMin=[]  KbOutMax=[]  KtOutMin=[]  KtOutMax=[]  IntegratorOutMin=[]  IntegratorOutMax=[]  FilterOutMin=[]  FilterOutMax=[]  SumI1OutMin=[]  SumI1OutMax=[]  SumI2OutMin=[]  SumI2OutMax=[]  SumI3OutMin=[]  SumI3OutMax=[]  SumI4OutMin=[]  SumI4OutMax=[]  SumDOutMin=[]  SumDOutMax=[]  DifferentiatorOutMin=[]  DifferentiatorOutMax=[]  FilterDiffOutCoefMin=[]  FilterDiffOutCoefMax=[]  ReciprocalOutMin=[]  ReciprocalOutMax=[]  SumDenOutMin=[]  SumDenOutMax=[]  SumNumOutMin=[]  SumNumOutMax=[]  DivideOutMin=[]  DivideOutMax=[]  UdiffTsProdOutMin=[]  UdiffTsProdOutMax=[]  NTsProdOutMin=[]  NTsProdOutMax=[]  UintegralTsProdOutMin=[]  UintegralTsProdOutMax=[]  UngainTsProdOutMin=[]  UngainTsProdOutMax=[]  IntegratorContinuousStateAttributes=''  IntegratorStateMustResolveToSignalObject=off  IntegratorRTWStateStorageClass=Auto  FilterContinuousStateAttributes=''  FilterStateMustResolveToSignalObject=off  FilterRTWStateStorageClass=Auto  ParallelPVariant=InternalParameters  IdealPVariant=Disabled  IVariant=InternalParameters  DVariant=Disabled  IntegratorVariant=Discrete  SatVariant=Disabled  AWVariant=Passthrough  PCopyVariant=Disabled  TRVariant=Disabled  FdbkBlocksVariant=Forward  IdealPFdbkVariant=Disabled  SatFdbkVariant=Disabled  DerivativeFilterVariant=Disabled  NVariant=Disabled  NCopyVariant=Disabled_SignalSpec  FilterICVariant=Disabled  IntegratorICVariant=InternalICs  ExternalResetVariant=Disabled  TRSumVariant=Passthrough  SumFdbkVariant=Disabled  SumVariant=Sum_PI  TsampFilterVariant=InternalTs  TsampNgainVariant=Passthrough  TsampIntegralVariant=Passthrough  ExternalSaturationOutDataTypeStr=Inherit: Same as second input
  PID Controller6 : slpidlib/PID Controller  Controller=PI  Form=Parallel  TimeDomain=Discrete-time  UseExternalTs=off  SampleTime=Ts  IntegratorMethod=Forward Euler  FilterMethod=Forward Euler  ControllerParametersSource=internal  P=10  I=30  D=0  UseFilter=on  N=100  TunerSelectOption=Transfer Function Based (PID Tuner App)  InitialConditionSource=internal  InitialConditionForIntegrator=0  InitialConditionForFilter=0  DifferentiatorICPrevScaledInput=0  ExternalReset=none  TrackingMode=off  Kt=1  LimitOutput=off  SatLimitsSource=internal  UpperSaturationLimit=inf  LowerSaturationLimit=-inf  LinearizeAsGain=on  AntiWindupMode=none  Kb=1  POutMin=[]  POutMax=[]  IOutMin=[]  IOutMax=[]  DOutMin=[]  DOutMax=[]  NOutMin=[]  NOutMax=[]  SumOutMin=[]  SumOutMax=[]  SaturationOutMin=[]  SaturationOutMax=[]  PParamMin=[]  PParamMax=[]  IParamMin=[]  IParamMax=[]  DParamMin=[]  DParamMax=[]  NParamMin=[]  NParamMax=[]  KbParamMin=[]  KbParamMax=[]  KtParamMin=[]  KtParamMax=[]  KbOutMin=[]  KbOutMax=[]  KtOutMin=[]  KtOutMax=[]  IntegratorOutMin=[]  IntegratorOutMax=[]  FilterOutMin=[]  FilterOutMax=[]  SumI1OutMin=[]  SumI1OutMax=[]  SumI2OutMin=[]  SumI2OutMax=[]  SumI3OutMin=[]  SumI3OutMax=[]  SumI4OutMin=[]  SumI4OutMax=[]  SumDOutMin=[]  SumDOutMax=[]  DifferentiatorOutMin=[]  DifferentiatorOutMax=[]  FilterDiffOutCoefMin=[]  FilterDiffOutCoefMax=[]  ReciprocalOutMin=[]  ReciprocalOutMax=[]  SumDenOutMin=[]  SumDenOutMax=[]  SumNumOutMin=[]  SumNumOutMax=[]  DivideOutMin=[]  DivideOutMax=[]  UdiffTsProdOutMin=[]  UdiffTsProdOutMax=[]  NTsProdOutMin=[]  NTsProdOutMax=[]  UintegralTsProdOutMin=[]  UintegralTsProdOutMax=[]  UngainTsProdOutMin=[]  UngainTsProdOutMax=[]  IntegratorContinuousStateAttributes=''  IntegratorStateMustResolveToSignalObject=off  IntegratorRTWStateStorageClass=Auto  FilterContinuousStateAttributes=''  FilterStateMustResolveToSignalObject=off  FilterRTWStateStorageClass=Auto  ParallelPVariant=InternalParameters  IdealPVariant=Disabled  IVariant=InternalParameters  DVariant=Disabled  IntegratorVariant=Discrete  SatVariant=Disabled  AWVariant=Passthrough  PCopyVariant=Disabled  TRVariant=Disabled  FdbkBlocksVariant=Forward  IdealPFdbkVariant=Disabled  SatFdbkVariant=Disabled  DerivativeFilterVariant=Disabled  NVariant=Disabled  NCopyVariant=Disabled_SignalSpec  FilterICVariant=Disabled  IntegratorICVariant=InternalICs  ExternalResetVariant=Disabled  TRSumVariant=Passthrough  SumFdbkVariant=Disabled  SumVariant=Sum_PI  TsampFilterVariant=InternalTs  TsampNgainVariant=Passthrough  TsampIntegralVariant=Passthrough  ExternalSaturationOutDataTypeStr=Inherit: Same as second input
  PID Controller7 : slpidlib/PID Controller  Controller=PI  Form=Parallel  TimeDomain=Discrete-time  UseExternalTs=off  SampleTime=Ts  IntegratorMethod=Forward Euler  FilterMethod=Forward Euler  ControllerParametersSource=internal  P=50  I=0  D=0  UseFilter=on  N=100  TunerSelectOption=Transfer Function Based (PID Tuner App)  InitialConditionSource=internal  InitialConditionForIntegrator=0  InitialConditionForFilter=0  DifferentiatorICPrevScaledInput=0  ExternalReset=none  TrackingMode=off  Kt=1  LimitOutput=off  SatLimitsSource=internal  UpperSaturationLimit=inf  LowerSaturationLimit=-inf  LinearizeAsGain=on  AntiWindupMode=none  Kb=1  POutMin=[]  POutMax=[]  IOutMin=[]  IOutMax=[]  DOutMin=[]  DOutMax=[]  NOutMin=[]  NOutMax=[]  SumOutMin=[]  SumOutMax=[]  SaturationOutMin=[]  SaturationOutMax=[]  PParamMin=[]  PParamMax=[]  IParamMin=[]  IParamMax=[]  DParamMin=[]  DParamMax=[]  NParamMin=[]  NParamMax=[]  KbParamMin=[]  KbParamMax=[]  KtParamMin=[]  KtParamMax=[]  KbOutMin=[]  KbOutMax=[]  KtOutMin=[]  KtOutMax=[]  IntegratorOutMin=[]  IntegratorOutMax=[]  FilterOutMin=[]  FilterOutMax=[]  SumI1OutMin=[]  SumI1OutMax=[]  SumI2OutMin=[]  SumI2OutMax=[]  SumI3OutMin=[]  SumI3OutMax=[]  SumI4OutMin=[]  SumI4OutMax=[]  SumDOutMin=[]  SumDOutMax=[]  DifferentiatorOutMin=[]  DifferentiatorOutMax=[]  FilterDiffOutCoefMin=[]  FilterDiffOutCoefMax=[]  ReciprocalOutMin=[]  ReciprocalOutMax=[]  SumDenOutMin=[]  SumDenOutMax=[]  SumNumOutMin=[]  SumNumOutMax=[]  DivideOutMin=[]  DivideOutMax=[]  UdiffTsProdOutMin=[]  UdiffTsProdOutMax=[]  NTsProdOutMin=[]  NTsProdOutMax=[]  UintegralTsProdOutMin=[]  UintegralTsProdOutMax=[]  UngainTsProdOutMin=[]  UngainTsProdOutMax=[]  IntegratorContinuousStateAttributes=''  IntegratorStateMustResolveToSignalObject=off  IntegratorRTWStateStorageClass=Auto  FilterContinuousStateAttributes=''  FilterStateMustResolveToSignalObject=off  FilterRTWStateStorageClass=Auto  ParallelPVariant=InternalParameters  IdealPVariant=Disabled  IVariant=InternalParameters  DVariant=Disabled  IntegratorVariant=Discrete  SatVariant=Disabled  AWVariant=Passthrough  PCopyVariant=Disabled  TRVariant=Disabled  FdbkBlocksVariant=Forward  IdealPFdbkVariant=Disabled  SatFdbkVariant=Disabled  DerivativeFilterVariant=Disabled  NVariant=Disabled  NCopyVariant=Disabled_SignalSpec  FilterICVariant=Disabled  IntegratorICVariant=InternalICs  ExternalResetVariant=Disabled  TRSumVariant=Passthrough  SumFdbkVariant=Disabled  SumVariant=Sum_PI  TsampFilterVariant=InternalTs  TsampNgainVariant=Passthrough  TsampIntegralVariant=Passthrough  ExternalSaturationOutDataTypeStr=Inherit: Same as second input
  Product{,1..5} (6 alike) : Product
  Relational Operator : RelationalOperator  OutDataTypeStr=boolean  RndMeth=Simplest
  Relational Operator1 : RelationalOperator  OutDataTypeStr=boolean  RndMeth=Simplest
  Relational Operator2 : RelationalOperator  OutDataTypeStr=boolean  RndMeth=Simplest
  Scope{2,9..12} (5 alike) : Scope  NumInputPorts=3
  Scope{3..4,6..7} (4 alike) : Scope  NumInputPorts=4
  Scope5 : Scope  NumInputPorts=6
  Scope8 : Scope  NumInputPorts=6
  Sine Wave1 : Sin  Commented=on  Frequency=2*pi*50  SampleTime=Ts
  Sine Wave2 : Sin  Commented=on  Frequency=2*pi*50  Phase=-120*2*pi/360  SampleTime=Ts
  Sine Wave3 : Sin  Commented=on  Frequency=2*pi*50  Phase=120*2*pi/360  SampleTime=Ts
  Sum{1..2,4..5,7..9,11,14..16} (11 alike) : Sum  Inputs=|+-
  Sum{3,6,10,12..13} (5 alike) : Sum  Inputs=|++
  Switch : Switch  Criteria=u2 > Threshold
  Triangle Generator : powerlib_meascontrol/Pulse & Signal Generators/Triangle Generator  Freq=10e3  Phase=90  Ts=0
  abc to Alpha-Beta-Zero : powerlib_meascontrol/Transformations/abc to Alpha-Beta-Zero  Commented=on
  dq0 to abc : powerlib_meascontrol/Transformations/dq0 to abc  Alignment=90 degrees behind phase A axis
  dq0 to abc1 : powerlib_meascontrol/Transformations/dq0 to abc  Alignment=90 degrees behind phase A axis
  Pulse : Outport
  wires:
  [Iq] -> Gain7/1
  Vq/1 -> [Vq]
  Iq/1 -> [Iq]
  Id/1 -> [Id]
  Vd/1 -> [Vd]
  [Id] -> Gain1/1
  [Id] -> Sum1/2, Scope7/2
  Enable/1 -> Product1/2, Product/2, Logical Operator7/2, Logical Operator3/2, Logical Operator4/2, Logical Operator5/2, Logical Operator8/2, Logical Operator6/2, Product3/2, Product2/2, Product4/2, Product5/2
  Product5/1 -> PID Controller6/1
  Sum16/1 -> Scope8/5, Product5/1
  Product4/1 -> PID Controller5/1
  Sum14/1 -> Product4/1
  Product3/1 -> PID Controller3/1
  Sum7/1 -> Product3/1, Scope4/3
  Product2/1 -> PID Controller4/1
  Sum11/1 -> Scope2/2, Product2/1
  Gain9/1 -> abc to Alpha-Beta-Zero/1
  Mux2/1 -> Gain9/1
  abc to Alpha-Beta-Zero/1 -> Alpha-Beta-Zero to dq0/1
  Sine Wave1/1 -> Mux2/1
  From33/1 -> Alpha-Beta-Zero to dq0/2
  Sine Wave2/1 -> Mux2/2
  Sine Wave3/1 -> Mux2/3
  Constant1/1 -> Scope6/1, Sum4/1
  Current/1 -> Sum1/1, Scope7/1
  dq0 to abc1/1 -> Switch/3
  dq0 to abc/1 -> Scope9/3, Switch/1
  [Vd] -> Sum7/2, Scope4/2
  Sum8/1 -> Sum9/1, Scope5/2
  Constant2/1 -> Sum11/1
  IqL/1 -> Sum12/2, Scope8/1
  PID Controller3/1 -> Sum8/1, Scope4/4
  Sum15/1 -> Mux1/1
  Gain7/1 -> Sum15/2
  Mux1/1 -> dq0 to abc1/1, Scope10/1
  [Id] -> Sum14/2
  Sum12/1 -> Sum13/1, Scope8/2
  PID Controller5/1 -> Scope5/6, Sum15/1
  PID Controller6/1 -> Scope8/6, Sum10/1
  [Id] -> Gain8/1
  Gain5/1 -> Sum9/2
  Gain6/1 -> Sum13/2, Scope8/3
  PID Controller4/1 -> Scope2/3, Sum12/1
  Gain8/1 -> Sum10/2
  [Iq] -> Sum16/2
  Sum13/1 -> Sum16/1, Scope8/4
  [Vq] -> Gain5/1
  Sum10/1 -> Mux1/2
  IdL/1 -> Sum8/2
  wt/1 -> dq0 to abc/2, Scope9/2, Scope10/2, dq0 to abc1/2
  [Vq] -> Scope2/1, Sum11/2
  Sum9/1 -> Sum14/1, Scope5/4
  [Vd] -> Gain6/1
  Constant3/1 -> Sum7/1, Scope4/1
  Alpha-Beta-Zero to dq0/1 -> Demux1/1
  mode/1 -> Switch/2
  Product1/1 -> PID Controller1/1
  [Iq] -> Gain/1, Scope6/2, Sum4/2
  Gain1/1 -> Sum5/2
  Sum4/1 -> Scope6/3, Product/1
  Sum2/1 -> Sum3/1, Scope11/1
  Sum5/1 -> Sum6/1, Scope12/1
  PID Controller2/1 -> Scope6/4, Sum5/1
  Mux/1 -> dq0 to abc/1, Scope9/1
  Sum1/1 -> Scope7/3, Product1/1
  Sum3/1 -> Scope11/3, Mux/1
  [Vq] -> Sum6/2, Scope12/2
  Sum6/1 -> Scope12/3, Mux/2
  Product/1 -> PID Controller2/1
  Gain/1 -> Sum2/2
  [Vd] -> Sum3/2, Scope11/2
  PID Controller1/1 -> Sum2/1, Scope7/4
  Divide2/1 -> Relational Operator2/1
  Gain4/1 -> Divide2/1
  Gain3/1 -> Divide1/1
  Divide1/1 -> Relational Operator1/1
  Vbus1/1 -> Divide/2, Divide1/2, Divide2/2
  Divide/1 -> Relational Operator/1, Scope3/2
  Gain2/1 -> Divide/1
  Logical Operator8/1 -> Bus Creator/1
  Logical Operator7/1 -> Bus Creator/2
  Logical Operator6/1 -> Bus Creator/3
  Logical Operator5/1 -> Bus Creator/4
  Logical Operator1/1 -> Logical Operator5/1
  Logical Operator4/1 -> Bus Creator/5
  Logical Operator2/1 -> Logical Operator3/1
  Logical Operator3/1 -> Bus Creator/6
  Bus Creator/1 -> Pulse/1
  Logical Operator/1 -> Logical Operator7/1, Scope3/4
  Demux3/1 -> Gain2/1
  Relational Operator/1 -> Logical Operator/1, Scope3/3, Logical Operator8/1
  Triangle Generator/1 -> Scope3/1, Relational Operator/2, Relational Operator1/2, Relational Operator2/2
  Relational Operator1/1 -> Logical Operator1/1, Logical Operator6/1
  Relational Operator2/1 -> Logical Operator2/1, Logical Operator4/1
  Switch/1 -> Demux3/1
  Demux3/3 -> Gain4/1
  Demux3/2 -> Gain3/1
